simulink model "pHSystem"  (R2016b)
settings: Solver=FixedStepDiscrete  StartTime=0.0  StopTime=inf  FixedStep=1  RelTol=1e-3  EnableMultiTasking=on
libraries: simulink x1
settings Model: ExtModeTrigDuration=2  Creator=rsjoshi1  LastModifiedBy=rsjoshi1
settings OptimizationCC: LifeSpan=Inf  MaxStackSize=64
settings DebuggingCC: SFUnexpectedBacktrackingDiag=warning  SFNoUnconditionalDefaultTransitionDiag=warning  SFExecutionAtInitializationDiag=none
settings HardwareCC: ProdBitPerPointer=32  ProdBitPerSizeT=32  ProdBitPerPtrDiffT=32  ProdLargestAtomicInteger=Long  ProdLargestAtomicFloat=Double  ProdWordSize=32  ProdHWDeviceType=ARM Compatible->ARM Cortex
settings RTWCC: SystemTargetFile=ert.tlc  HardwareBoard=Arduino Due  TLCOptions=-aInlineSetEventsForThisBaseRateFcn=TLC_FALSE -aSuppressMultiTaskScheduler=TLC_FALSE -aRateBasedStepFcn=1  TemplateMakefile=ert_default_tmf  Description=Embedded Coder  GenerateReport=on  Toolchain=Arduino ARM v1.6.7  BuildConfiguration=Faster Runs  IncludeHyperlinkInReport=on  LaunchReport=on  GenerateTraceInfo=on  GenerateTraceReport=on  GenerateTraceReportSl=on  GenerateTraceReportSf=on  GenerateTraceReportEml=on
settings CodeAppCC: ForceParamTrailComments=on  IgnoreCustomStorageClasses=off  OperatorAnnotations=on  SimulinkDataObjDesc=on  SFDataObjDesc=on  MATLABFcnDesc=on  InsertBlockDesc=on  MATLABSourceComments=on
settings ERTTargetCC: SupportContinuousTime=on  SupportVariableSizeSignals=on
settings ConfigComp: CovMetricSettings=dw  CovHtmlReporting=on  CovSaveCumulativeToWorkspaceVar=on  CovSaveSingleToWorkspaceVar=on  CovExternalEMLEnable=off

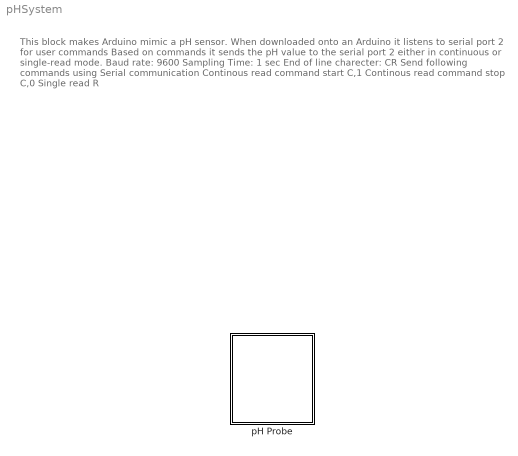
== system pHSystem ==
  note: This block makes Arduino mimic a pH sensor.
      | When downloaded onto an Arduino it listens to serial port 2 for user commands
      | Based on commands it sends the pH value to the serial port 2 either in continuous or single-read mode.
      |
      | Baud rate: 9600
      | Sampling Time: 1 sec
      | End of line charecter: CR
      |
      | Send following commands using Serial communication
      |
      | Continous read command start C,1
      | Continous read command stop C,0
      | Single read R
  pH Probe : Subsystem  Description=pH probe
      mask Display: disp('pH Sensor')

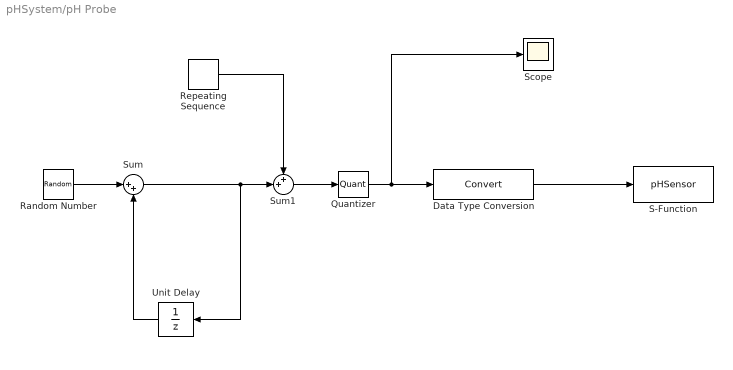
== system pHSystem/pH Probe ==
  Data Type Conversion : DataTypeConversion
  Quantizer : Quantizer  QuantizationInterval=0.04
  Random Number : RandomNumber  Variance=0.00005  SampleTime=1
  Repeating Sequence : simulink/Sources/Repeating Sequence  rep_seq_t=[0 0.2]  rep_seq_y=[0 0.2]
  S-Function : S-Function  FunctionName=pHSensor  Parameters=int8(2)  SFunctionModules=pHSensor_wrapper  SFunctionDeploymentMode=off  EnableBusSupport=off
  Scope : Scope
  Sum : Sum  Inputs=|++
  Sum1 : Sum  Inputs=++|
  Unit Delay : UnitDelay  InitialCondition=6+2*rand
  wires:
  Data Type Conversion/1 -> S-Function/1
  Random Number/1 -> Sum/1
  Sum/1 -> Sum1/2, Unit Delay/1
  Unit Delay/1 -> Sum/2
  Quantizer/1 -> Scope/1, Data Type Conversion/1
  Sum1/1 -> Quantizer/1
  Repeating Sequence/1 -> Sum1/1
